simulink model "automatic_transmission_system_v2"  (R2021a)
settings: Solver=ode15s  StartTime=0.0  StopTime=100  FixedStep=0.1  RelTol=1e-3  EnableMultiTasking=on
settings Model: Creator=glembrez  LastModifiedBy=gabin
settings SolverCC: AlgebraicLoopSolver=TrustRegion  AutoInsertRateTranBlk=on
settings DataIOCC: LimitDataPoints=on
settings OptimizationCC: LifeSpan=inf
settings DebuggingCC: AllowSymbolicDim=off  SFUnexpectedBacktrackingDiag=warning  SFNoUnconditionalDefaultTransitionDiag=warning  SFExecutionAtInitializationDiag=none  ArithmeticOperatorsInVariantConditions=warning
settings SFSimCC: SimUseLocalCustomCode=off  CustomCodeUndefinedFunction=UseInterfaceOnly
settings RTWCC: RTWUseLocalCustomCode=off
settings CodeAppCC: StateflowObjectComments=on
settings GRTTargetCC: TargetLangStandard=C89/C90 (ANSI)
settings ConfigComp: CovMetricSettings=dw  CovSaveCumulativeToWorkspaceVar=on  CovSaveSingleToWorkspaceVar=on  CovExternalEMLEnable=off  CovSFcnEnable=off

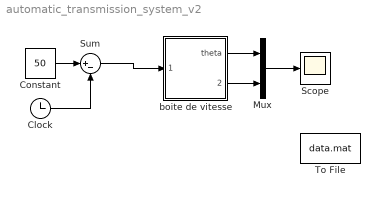
== system automatic_transmission_system_v2 ==
  Clock : Clock
  Constant : Constant  Value=50
  Mux : Mux  Inputs=2
  Scope : Scope
  Sum : Sum  Inputs=|+-
  To File : ToFile  Filename=data.mat  MatrixName=X  SaveFormat=Timeseries
  boite de vitesse : Stateflow chart  TreatAsAtomicUnit=on
  wires:
  Mux/1 -> Scope/1
  boite de vitesse/1(theta) -> Mux/1
  boite de vitesse/2(omega) -> Mux/2
  Constant/1 -> Sum/1
  Clock/1 -> Sum/2
  Sum/1 -> boite de vitesse/1(conductor)

== stateflow chart automatic_transmission_system_v2/boite de vitesse ==
  settings: updateMethod=CONTINUOUS
  state Transmission [parallel]
    %Les valeurs de transition entre UP et DOWN
    %sont optimisées pour les conditions décrites dans l'article
    %les enlever ?
    settings: executionOrder=1
    state Neutral
      during :
      theta_dot = 0;
      omega_dot = 0;
    state Gear1_DOWN
      during :
      theta_dot = omega;
      omega_dot = d*0.99*exp(-(omega-a1)^2/64)+0.01;
    state Gear1_UP
      during :
      theta_dot = omega;
      omega_dot = u*0.99*exp(-((omega-a1)^2)/64)+0.01;
    state Gear2_DOWN
      during :
      theta_dot = omega;
      omega_dot = d*0.99*exp(-(omega-a2)^2/64)+0.01;
    state Gear2_UP
      during :
      theta_dot = omega;
      omega_dot = u*0.99*exp(-((omega-a2)^2)/64)+0.01;
    state Gear3_DOWN
      during :
      theta_dot = omega;
      omega_dot = d*0.99*exp(-(omega-a3)^2/64)+0.01;
    state Gear3_UP
      during :
      theta_dot = omega;
      omega_dot = u*0.99*exp(-((omega-a3)^2)/64)+0.01;
    (default) -> Neutral
    Gear1_DOWN -> Neutral [order 1] : [after(5,sec)...
        | &&-epsilon<=omega...
        | &&epsilon>= omega...
        | &&in(Conductor.deaccelerating)]
    Neutral -> Gear1_UP : [-epsilon<=omega...
        | &&epsilon>= omega...
        | &&in(Conductor.accelerating)]
    Gear1_DOWN -> Gear1_UP [order 2] : [after(5,sec)...
        | &&-epsilon<=omega...
        | &&epsilon>= omega...
        | &&in(Conductor.accelerating)]
    Gear1_UP -> Gear1_DOWN [order 2] : [after(5,sec)...
        | &&1.31<=omega...
        | &&omega<=16.7...
        | &&in(Conductor.deaccelerating)]
    Gear2_DOWN -> Gear1_DOWN [order 1] : [after(5,sec)...
        | &&1.31<=omega...
        | &&omega<=16.70]
    Gear1_UP -> Gear2_UP [order 1] : [after(5,sec)...
        | &&13.29<=omega...
        | &&omega<=23.42]
    Gear2_DOWN -> Gear2_UP [order 2] : [after(5,sec)...
        | &&13.29<=omega...
        | &&omega<=23.42...
        | &&in(Conductor.accelerating)]
    Gear2_UP -> Gear2_DOWN [order 2] : [after(5,sec)...
        | &&26.7-epsilon<=omega...
        | &&epsilon+26.7>= omega...
        | &&in(Conductor.deaccelerating)]
    Gear3_DOWN -> Gear2_DOWN [order 1] : [after(5,sec)...
        | &&16.58<=omega...
        | &&omega<=26.7]
    Gear2_UP -> Gear3_UP [order 1] : [after(5,sec)...
        | &&26.7<=omega...
        | &&omega<=33.42]
    Gear3_DOWN -> Gear3_UP [order 2] : [after(5,sec)...
        | &&23.29<=omega...
        | &&omega<=33.42...
        | &&in(Conductor.accelerating)]
    Gear3_UP -> Gear3_DOWN : [omega>=36.7...
        | &&in(Conductor.deaccelerating)]
  state Conductor [parallel]
    settings: executionOrder=2
    state accelerating
    state deaccelerating
    (default) -> accelerating
    accelerating -> deaccelerating : [conductor<0]
    deaccelerating -> accelerating : [conductor>=0]
  data: theta output =0; omega output =0; d local =-1; u local =1; a1 local =10; a2 local =20; a3 local =30; thetamax local =1700; epsilon local =1; conductor input
  data theta settings: updateMethod=SF_CONTINUOUS_TIME_DATA
  data omega settings: updateMethod=SF_CONTINUOUS_TIME_DATA
